simulink model "IN_OUT_Test"  (Simulink 7.6)
settings: Solver=FixedStepDiscrete  SolverMode=SingleTasking  StartTime=0.0  StopTime=20  FixedStep=1  RelTol=1e-3
libraries: simulink x17
settings Model: Creator=jordan  LastModifiedBy=jordan
settings DataIOCC: LimitDataPoints=off  SaveOutput=off  SignalLogging=off  DSMLogging=off  SaveTime=off

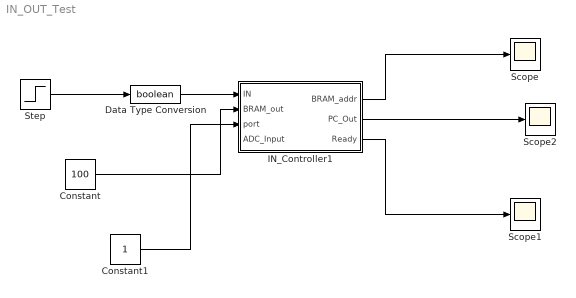
== system IN_OUT_Test ==
  Constant : Constant  Value=100  OutDataTypeStr=uint8
  Constant1 : Constant  OutDataTypeStr=fixdt(0,5,0)
  Data Type Conversion : DataTypeConversion  OutDataTypeStr=boolean
  IN_Controller1 : Subsystem
  Scope : Scope
  Scope1 : Scope
  Scope2 : Scope
      settings: SaveName=ScopeData6
  Step : Step  Time=5  SampleTime=1
  wires:
  Step/1 -> Data Type Conversion/1
  IN_Controller1/1(BRAM_addr) -> Scope/1
  IN_Controller1/3(Ready) -> Scope1/1
  Data Type Conversion/1 -> IN_Controller1/1(IN)
  IN_Controller1/2(PC_Out) -> Scope2/1
  Constant/1 -> IN_Controller1/2(BRAM_out)
  Constant1/1 -> IN_Controller1/3(port)

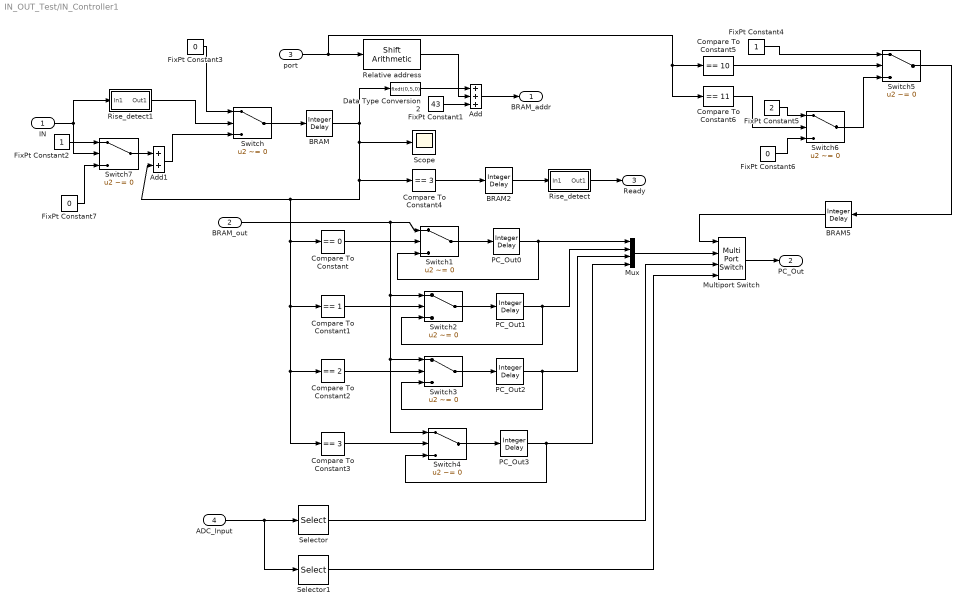
== system IN_OUT_Test/IN_Controller1 ==
  IN : Inport  OutDataTypeStr=boolean
  BRAM_out : Inport  Port=2  OutDataTypeStr=uint8
  port : Inport  Port=3  OutDataTypeStr=fixdt(0,5,0)
  ADC_Input : Inport  Port=4  OutDataTypeStr=uint8  PortDimensions=8
  Add : Sum  Inputs=+++  AccumDataTypeStr=fixdt(0,11,0)  OutDataTypeStr=fixdt(0,11,0)
  Add1 : Sum  AccumDataTypeStr=fixdt(0,2,0)  OutDataTypeStr=fixdt(0,2,0)  SaturateOnIntegerOverflow=on
  BRAM : simulink/Discrete/Integer Delay  NumDelays=2  vinit=0.0  samptime=0
  BRAM2 : simulink/Discrete/Integer Delay  NumDelays=1  vinit=0.0  samptime=0
  BRAM5 : simulink/Discrete/Integer Delay  NumDelays=1  vinit=0.0  samptime=0
  Compare To Constant : simulink/Logic and Bit Operations/Compare To Constant  SystemSampleTime=-1  relop===  const=0  LogicOutDataTypeMode=boolean
  Compare To Constant1 : simulink/Logic and Bit Operations/Compare To Constant  SystemSampleTime=-1  relop===  const=1  LogicOutDataTypeMode=boolean
  Compare To Constant2 : simulink/Logic and Bit Operations/Compare To Constant  SystemSampleTime=-1  relop===  const=2  LogicOutDataTypeMode=boolean
  Compare To Constant3 : simulink/Logic and Bit Operations/Compare To Constant  SystemSampleTime=-1  relop===  const=3  LogicOutDataTypeMode=boolean
  Compare To Constant4 : simulink/Logic and Bit Operations/Compare To Constant  SystemSampleTime=-1  relop===  const=3  LogicOutDataTypeMode=boolean
  Compare To Constant5 : simulink/Logic and Bit Operations/Compare To Constant  SystemSampleTime=-1  relop===  const=10  LogicOutDataTypeMode=boolean
  Compare To Constant6 : simulink/Logic and Bit Operations/Compare To Constant  SystemSampleTime=-1  relop===  const=11  LogicOutDataTypeMode=boolean
  Data Type Conversion2 : DataTypeConversion  OutDataTypeStr=fixdt(0,5,0)
  FixPt Constant1 : Constant  DisableCoverage=on  Value=43  OutDataTypeStr=fixdt(0,11,0)
  FixPt Constant2 : Constant  DisableCoverage=on  OutDataTypeStr=fixdt(0,2,0)
  FixPt Constant3 : Constant  DisableCoverage=on  Value=0  OutDataTypeStr=fixdt(0,2,0)
  FixPt Constant4 : Constant  DisableCoverage=on  OutDataTypeStr=fixdt(0,2,0)
  FixPt Constant5 : Constant  DisableCoverage=on  Value=2  OutDataTypeStr=fixdt(0,2,0)
  FixPt Constant6 : Constant  DisableCoverage=on  Value=0  OutDataTypeStr=fixdt(0,2,0)
  FixPt Constant7 : Constant  DisableCoverage=on  Value=0  OutDataTypeStr=fixdt(0,2,0)
  Multiport Switch : MultiPortSwitch  DataPortOrder=Zero-based contiguous  zeroidx=on
  Mux : Mux
  PC_Out{0..3} (4 alike) : simulink/Discrete/Integer Delay  NumDelays=1  vinit=0.0  samptime=-1
  Relative address : simulink/Logic and Bit Operations/Shift Arithmetic  SystemSampleTime=-1  nBitShiftRight=-2  nBinPtShiftRight=0
  Rise_detect : Subsystem
  Rise_detect1 : Subsystem
  Scope : Scope
      settings: SaveName=ScopeData2
  Selector : Selector  InputPortWidth=8  IndexOptions=Index vector (dialog)  Indices=1:4  OutputSizes=1
  Selector1 : Selector  InputPortWidth=8  IndexOptions=Index vector (dialog)  Indices=5:8  OutputSizes=1
  Switch{,1..7} (8 alike) : Switch  Criteria=u2 ~= 0
  BRAM_addr : Outport
  PC_Out : Outport  Port=2  OutDataTypeStr=uint8  PortDimensions=4
  Ready : Outport  Port=3
  wires:
  Rise_detect/1(Out1) -> Ready/1
  BRAM/1 -> Data Type Conversion2/1, Compare To Constant4/1, Add1/2, Compare To Constant/1, Compare To Constant1/1, Compare To Constant2/1, Compare To Constant3/1, Scope/1
  Add/1 -> BRAM_addr/1
  Data Type Conversion2/1 -> Add/1
  FixPt Constant1/1 -> Add/3
  Switch/1 -> BRAM/1
  Add1/1 -> Switch/3
  FixPt Constant2/1 -> Switch7/1
  Switch1/1 -> PC_Out0/1
  PC_Out0/1 -> Switch1/3, Mux/1
  Compare To Constant/1 -> Switch1/2
  Switch2/1 -> PC_Out1/1
  PC_Out1/1 -> Switch2/3, Mux/2
  Compare To Constant1/1 -> Switch2/2
  Switch3/1 -> PC_Out2/1
  PC_Out2/1 -> Switch3/3, Mux/3
  Compare To Constant2/1 -> Switch3/2
  Switch4/1 -> PC_Out3/1
  PC_Out3/1 -> Switch4/3, Mux/4
  Compare To Constant3/1 -> Switch4/2
  BRAM_out/1 -> Switch1/1, Switch2/1, Switch3/1, Switch4/1
  Relative address/1 -> Add/2
  port/1 -> Relative address/1, Compare To Constant5/1, Compare To Constant6/1
  IN/1 -> Switch7/2, Rise_detect1/1(In1)
  Mux/1 -> Multiport Switch/2
  Rise_detect1/1(Out1) -> Switch/2
  FixPt Constant3/1 -> Switch/1
  Compare To Constant4/1 -> BRAM2/1
  BRAM2/1 -> Rise_detect/1(In1)
  Multiport Switch/1 -> PC_Out/1
  Selector/1 -> Multiport Switch/3
  ADC_Input/1 -> Selector/1, Selector1/1
  Selector1/1 -> Multiport Switch/4
  Compare To Constant5/1 -> Switch5/2
  Compare To Constant6/1 -> Switch6/2
  FixPt Constant4/1 -> Switch5/1
  FixPt Constant5/1 -> Switch6/1
  FixPt Constant6/1 -> Switch6/3
  Switch6/1 -> Switch5/3
  Switch5/1 -> BRAM5/1
  Switch7/1 -> Add1/1
  FixPt Constant7/1 -> Switch7/3
  BRAM5/1 -> Multiport Switch/1

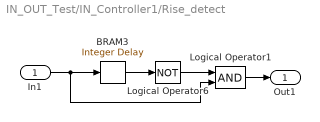
== system IN_OUT_Test/IN_Controller1/Rise_detect ==
  In1 : Inport
  BRAM3 : simulink/Discrete/Integer Delay  NumDelays=1  vinit=0.0  samptime=-1
  Logical Operator1 : Logic  AllPortsSameDT=off  OutDataTypeStr=boolean
  Logical Operator6 : Logic  Operator=NOT  AllPortsSameDT=off  OutDataTypeStr=boolean
  Out1 : Outport
  wires:
  Logical Operator6/1 -> Logical Operator1/1
  BRAM3/1 -> Logical Operator6/1
  In1/1 -> BRAM3/1, Logical Operator1/2
  Logical Operator1/1 -> Out1/1

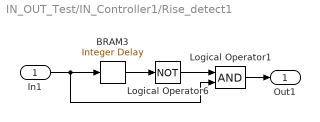
== system IN_OUT_Test/IN_Controller1/Rise_detect1 ==
  In1 : Inport
  BRAM3 : simulink/Discrete/Integer Delay  NumDelays=1  vinit=0.0  samptime=-1
  Logical Operator1 : Logic  AllPortsSameDT=off  OutDataTypeStr=boolean
  Logical Operator6 : Logic  Operator=NOT  AllPortsSameDT=off  OutDataTypeStr=boolean
  Out1 : Outport
  wires:
  Logical Operator1/1 -> Out1/1
  In1/1 -> Logical Operator1/2, BRAM3/1
  BRAM3/1 -> Logical Operator6/1
  Logical Operator6/1 -> Logical Operator1/1
